simulink model "goertzel_algorithm1"  (R2021b)
settings: Solver=FixedStepAuto  StartTime=0.0  StopTime=100.0  FixedStep=0.001  RelTol=1e-3
libraries: hdlsllib x2, commrandsrc3 x1, simulink x1
settings Model: Creator=caccolillo  LastModifiedBy=caccolillo

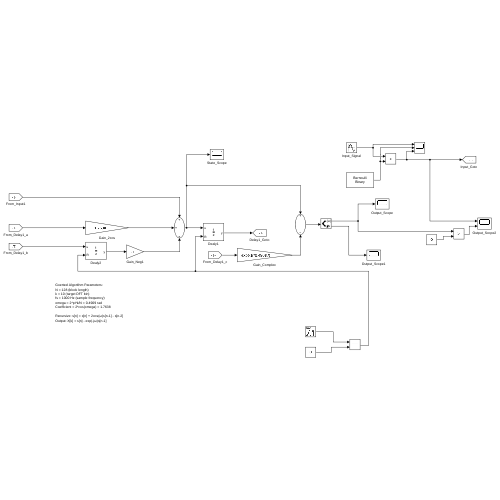
[thumbnail: Simulink's stored preview of the top-level diagram]
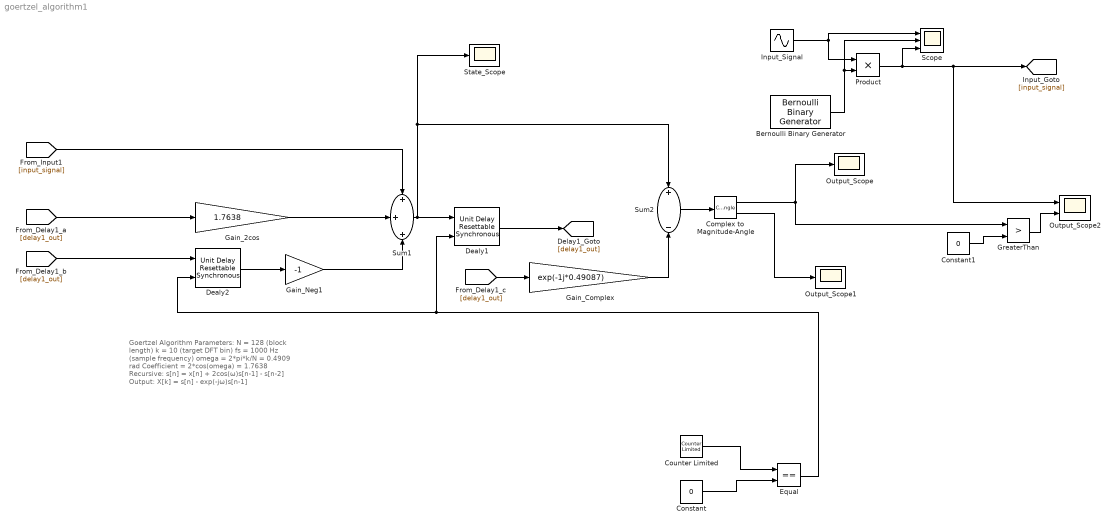
== system goertzel_algorithm1 ==
  note: Goertzel Algorithm Parameters:
      | N = 128 (block length)
      | k = 10 (target DFT bin)
      | fs = 1000 Hz (sample frequency)
      | omega = 2*pi*k/N = 0.4909 rad
      | Coefficient = 2*cos(omega) = 1.7638
      |
      | Recursive: s[n] = x[n] + 2cos(ω)s[n-1] - s[n-2]
      | Output: X[k] = s[n] - exp(-jω)s[n-1]
  Bernoulli Binary Generator : commrandsrc3/Bernoulli Binary Generator  ProbabilityOfZero=0.5  SeedSource=Auto  Seed=0  SampleTime=1  SamplesPerFrame=1  OutputDataType=double  SimulateUsing=Interpreted execution
  Complex to Magnitude-Angle : ComplexToMagnitudeAngle
  Constant : Constant  Value=0
  Constant1 : Constant  Value=0
  Counter Limited : simulink/Sources/Counter Limited  uplimit=128  tsamp=0.001
  Dealy1 : hdlsllib/Discrete/Unit Delay Resettable Synchronous  InitialCondition=0.0  SampleTime=-1
      settings: SourceProductBaseCode=SL
  Dealy2 : hdlsllib/Discrete/Unit Delay Resettable Synchronous  InitialCondition=0.0  SampleTime=-1
      settings: SourceProductBaseCode=SL
  Equal : RelationalOperator  Operator===  OutDataTypeStr=boolean  RndMeth=Simplest
  Gain_2cos : Gain  Gain=1.7638
  Gain_Complex : Gain  Gain=exp(-1j*0.49087)
  Gain_Neg1 : Gain  Gain=-1
  GreaterThan : RelationalOperator  Operator=>  OutDataTypeStr=boolean  RndMeth=Simplest
  Input_Signal : Sin  Frequency=2*pi*50  SampleTime=0.001
  Output_Scope : Scope
  Output_Scope1 : Scope
  Output_Scope2 : Scope  NumInputPorts=2
  Product : Product
  Scope : Scope  NumInputPorts=3
  State_Scope : Scope
  Sum1 : Sum  Inputs=+++
  Sum2 : Sum  Inputs=+-
  wires:
  [input_signal] -> Sum1/1
  [delay1_out] -> Gain_2cos/1
  Gain_2cos/1 -> Sum1/2
  [delay1_out] -> Dealy2/1
  Dealy2/1 -> Gain_Neg1/1
  Gain_Neg1/1 -> Sum1/3
  Sum1/1 -> Sum2/1, State_Scope/1, Dealy1/1
  Dealy1/1 -> [delay1_out]
  [delay1_out] -> Gain_Complex/1
  Gain_Complex/1 -> Sum2/2
  Sum2/1 -> Complex to Magnitude-Angle/1
  Input_Signal/1 -> Product/1, Scope/1
  Bernoulli Binary Generator/1 -> Scope/2, Product/2
  Product/1 -> Output_Scope2/1, [input_signal], Scope/3
  Complex to Magnitude-Angle/1 -> GreaterThan/1, Output_Scope/1
  Complex to Magnitude-Angle/2 -> Output_Scope1/1
  Counter Limited/1 -> Equal/1
  Constant/1 -> Equal/2
  Equal/1 -> Dealy2/2, Dealy1/2
  GreaterThan/1 -> Output_Scope2/2
  Constant1/1 -> GreaterThan/2
